simulink model "EGR_CAN"  (R2013b)
settings: Solver=FixedStepDiscrete  StartTime=0.0  StopTime=0.5  FixedStep=Ts  RelTol=1e-3
values from neighbouring files (symbols this model uses):
  C_STEPM_ELEC_TIM_COEFF = Simulink.Parameter    [EGR_CAN_Model_Init.m]
  K_EGR_CAN_ACT_DC_COMP = Simulink.Parameter    [EGR_CAN_Model_Init.m]
  K_EGR_CAN_ACT_POS_MAX = Simulink.Parameter    [EGR_CAN_Model_Init.m]
  K_EGR_CAN_ACT_POS_MIN = Simulink.Parameter    [EGR_CAN_Model_Init.m]
  K_EGR_CAN_TARGET_POS_MAX = Simulink.Parameter    [EGR_CAN_Model_Init.m]
  K_EGR_CAN_TARGET_POS_MIN = Simulink.Parameter    [EGR_CAN_Model_Init.m]
  K_PID_D_TERM = Simulink.Parameter    [EGR_CAN_Model_Init.m]
  K_PID_I_TERM = Simulink.Parameter    [EGR_CAN_Model_Init.m]
  K_PID_P_TERM = Simulink.Parameter    [EGR_CAN_Model_Init.m]
  K_STEPM_DAMPING_COEFF = Simulink.Parameter    [EGR_CAN_Model_Init.m]
  K_STEPM_INERTIA = Simulink.Parameter    [EGR_CAN_Model_Init.m]
  K_STEPM_SELF_DAMPING_COEFF = Simulink.Parameter    [EGR_CAN_Model_Init.m]
  K_STEPM_STEP_NUM = Simulink.Parameter    [EGR_CAN_Model_Init.m]
  K_STEPM_TF = Simulink.Parameter    [EGR_CAN_Model_Init.m]
  Ts = 1e-4    (= 0.0001)    [EGR_CAN_Model_Init.m]
undefined symbols (not defined in the file or in its folder): DiscIntNeverNeededParam
libraries: simulink x1
settings Model: Creator=Administrator  LastModifiedBy=TTI1783
settings OptimizationCC: InlineParams=on  UseFloatMulNetSlope=on  UseSpecifiedMinMax=on  InlineInvariantSignals=on  EnhancedBackFolding=on  ZeroExternalMemoryAtStartup=off  ZeroInternalMemoryAtStartup=off  EfficientFloat2IntCast=on  OptimizeModelRefInitCode=on  LifeSpan=1  MaxStackSize=64
settings DebuggingCC: MergeDetectMultiDrivingBlocksExec=error
settings HardwareCC: ProdLargestAtomicInteger=Long  ProdLargestAtomicFloat=Double  ProdIntDivRoundTo=Floor  ProdEndianess=LittleEndian  ProdHWDeviceType=ARM Compatible->ARM Cortex
settings RTWCC: SystemTargetFile=ert.tlc  GenCodeOnly=on  GenerateMakefile=off  TemplateMakefile=ert_default_tmf  Description=Embedded Coder  GenerateReport=on  ProcessScript=ert_make_rtw_hook  Toolchain=GNU Tools for ARM Embedded Processors  IncludeHyperlinkInReport=on  LaunchReport=on  GenerateTraceInfo=on  GenerateTraceReport=on  GenerateTraceReportSl=on  GenerateTraceReportSf=on  GenerateTraceReportEml=on  RTWCompilerOptimization=On
settings CodeAppCC: ForceParamTrailComments=on  IgnoreCustomStorageClasses=off  OperatorAnnotations=on  SimulinkDataObjDesc=on  SFDataObjDesc=on  MATLABFcnDesc=on  InsertBlockDesc=on  MATLABSourceComments=on  EnableCustomComments=on  ReqsInCode=on
settings ERTTargetCC: CodeReplacementLibrary=ANSI_C  GenerateSampleERTMain=on  IncludeMdlTerminateFcn=off  CombineSignalStateStructs=on  SuppressErrorStatus=on  SupportNonFinite=off  InlinedParameterPlacement=NonHierarchical  ERTCustomFileTemplate=example_file_process.tlc  ConvertIfToSwitch=on  SuppressUnreachableDefaultCases=on

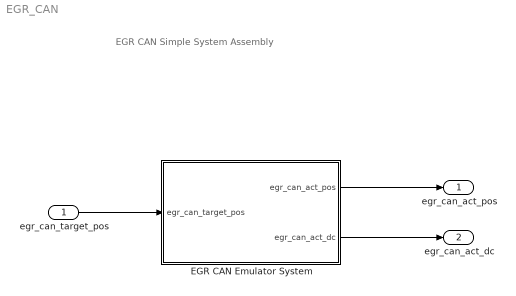
== system EGR_CAN ==
  note: EGR CAN Simple System Assembly
  egr_can_target_pos : Inport
  EGR CAN Emulator System : Subsystem
  egr_can_act_pos : Outport
  egr_can_act_dc : Outport  Port=2
  wires:
  EGR CAN Emulator System/1(egr_can_act_pos) -> egr_can_act_pos/1
  egr_can_target_pos/1 -> EGR CAN Emulator System/1(egr_can_target_pos)
  EGR CAN Emulator System/2(egr_can_act_dc) -> egr_can_act_dc/1

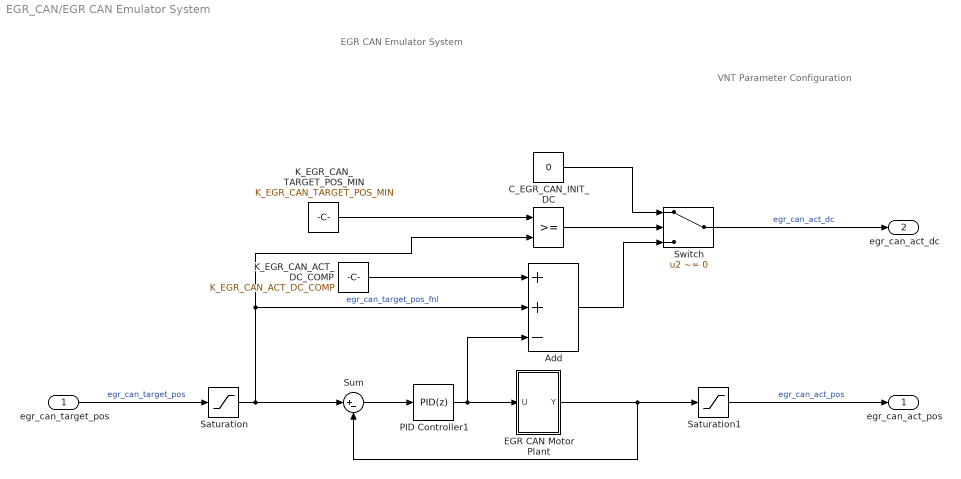
== system EGR_CAN/EGR CAN Emulator System ==
  note: VNT Parameter
      | Configuration
  note: EGR CAN Emulator System
  egr_can_target_pos : Inport
  " " : RelationalOperator  OutDataTypeStr=boolean
  Add : Sum  Inputs=++-
  C_EGR_CAN_INIT_DC : Constant  Value=0
  EGR CAN Motor Plant : Subsystem
  K_EGR_CAN_ACT_DC_COMP : Constant  Value=K_EGR_CAN_ACT_DC_COMP
  K_EGR_CAN_TARGET_POS_MIN : Constant  Value=K_EGR_CAN_TARGET_POS_MIN
  PID Controller1 : simulink/Continuous/PID Controller  Controller=PID  TimeDomain=Discrete-time  SampleTime=Ts  IntegratorMethod=Forward Euler  FilterMethod=Forward Euler  Form=Ideal  P=K_PID_P_TERM  I=K_PID_I_TERM  D=K_PID_D_TERM  N=100  InitialConditionSource=internal  InitialConditionForIntegrator=0  InitialConditionForFilter=0  ExternalReset=none  LimitOutput=off  UpperSaturationLimit=inf  LowerSaturationLimit=-inf  LinearizeAsGain=on  AntiWindupMode=none  Kb=1  TrackingMode=off  Kt=1  PParamMin=[]  PParamMax=[]  IParamMin=[]  IParamMax=[]  DParamMin=[]  DParamMax=[]  NParamMin=[]  NParamMax=[]  KbParamMin=[]  KbParamMax=[]  KtParamMin=[]  KtParamMax=[]  POutMin=[]  POutMax=[]  IOutMin=[]  IOutMax=[]  DOutMin=[]  DOutMax=[]  NOutMin=[]  NOutMax=[]  KbOutMin=[]  KbOutMax=[]  KtOutMin=[]  KtOutMax=[]  IntegratorOutMin=[]  IntegratorOutMax=[]  FilterOutMin=[]  FilterOutMax=[]  SumOutMin=[]  SumOutMax=[]  SumI1OutMin=[]  SumI1OutMax=[]  SumI2OutMin=[]  SumI2OutMax=[]  SumI3OutMin=[]  SumI3OutMax=[]  SumDOutMin=[]  SumDOutMax=[]  SaturationOutMin=[]  SaturationOutMax=[]  IntegratorContinuousStateAttributes=''  IntegratorStateMustResolveToSignalObject=off  IntegratorRTWStateStorageClass=Auto  FilterContinuousStateAttributes=''  FilterStateMustResolveToSignalObject=off  FilterRTWStateStorageClass=Auto
  Saturation : Saturate  UpperLimit=K_EGR_CAN_TARGET_POS_MAX  LowerLimit=K_EGR_CAN_TARGET_POS_MIN
  Saturation1 : Saturate  UpperLimit=K_EGR_CAN_ACT_POS_MAX  LowerLimit=K_EGR_CAN_ACT_POS_MIN
  Sum : Sum  Inputs=|+-
  Switch : Switch  Criteria=u2 ~= 0
  egr_can_act_pos : Outport
  egr_can_act_dc : Outport  Port=2
  wires:
  egr_can_target_pos/1 -> Saturation/1  "egr_can_target_pos"
  PID Controller1/1 -> Add/3, EGR CAN Motor Plant/1(U)
  Sum/1 -> PID Controller1/1
  Saturation1/1 -> egr_can_act_pos/1  "egr_can_act_pos"
  EGR CAN Motor Plant/1(Y) -> Saturation1/1, Sum/2
  Saturation/1 -> Add/2, " "/2, Sum/1  "egr_can_target_pos_fnl"
  K_EGR_CAN_ACT_DC_COMP/1 -> Add/1
  Add/1 -> Switch/3
  Switch/1 -> egr_can_act_dc/1  "egr_can_act_dc"
  " "/1 -> Switch/2
  C_EGR_CAN_INIT_DC/1 -> Switch/1
  K_EGR_CAN_TARGET_POS_MIN/1 -> " "/1

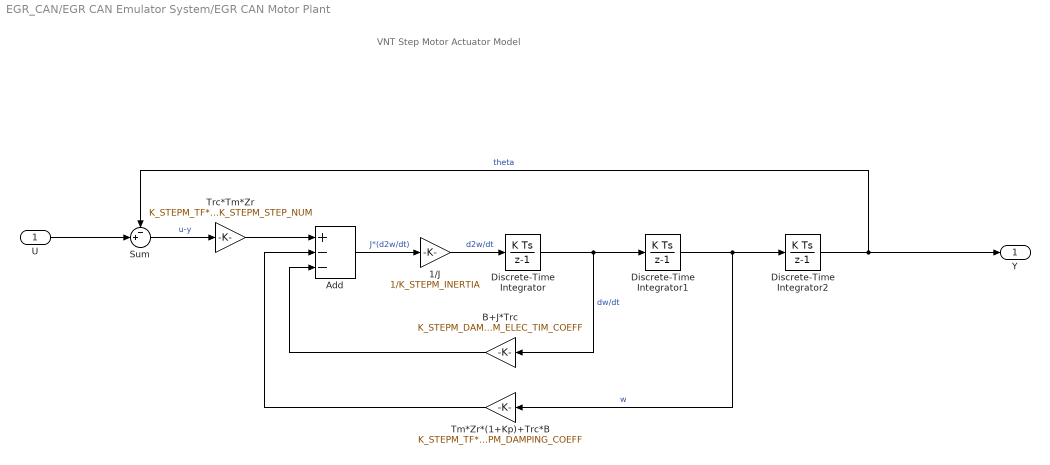
== system EGR_CAN/EGR CAN Emulator System/EGR CAN Motor Plant ==
  note: VNT Step Motor Actuator Model
  U : Inport
  1/J : Gain  Gain=1/K_STEPM_INERTIA
  Add : Sum  Inputs=+--
  B+J*Trc : Gain  Gain=K_STEPM_DAMPING_COEFF+K_STEPM_INERTIA*C_STEPM_ELEC_TIM_COEFF
  Discrete-Time Integrator : DiscreteIntegrator  SampleTime=Ts  ICPrevOutput=DiscIntNeverNeededParam  ICPrevScaledInput=DiscIntNeverNeededParam
  Discrete-Time Integrator1 : DiscreteIntegrator  SampleTime=Ts  ICPrevOutput=DiscIntNeverNeededParam  ICPrevScaledInput=DiscIntNeverNeededParam
  Discrete-Time Integrator2 : DiscreteIntegrator  SampleTime=Ts  ICPrevOutput=DiscIntNeverNeededParam  ICPrevScaledInput=DiscIntNeverNeededParam
  Sum : Sum  Inputs=-+|
  Tm*Zr*(1+Kp)+Trc*B : Gain  Gain=K_STEPM_TF*K_STEPM_STEP_NUM*(1+K_STEPM_SELF_DAMPING_COEFF)+C_STEPM_ELEC_TIM_COEFF*K_STEPM_DAMPING_COEFF
  Trc*Tm*Zr : Gain  Gain=K_STEPM_TF*C_STEPM_ELEC_TIM_COEFF*K_STEPM_STEP_NUM
  Y : Outport
  wires:
  B+J*Trc/1 -> Add/3
  Add/1 -> 1/J/1  "J*(d2w/dt)"
  Trc*Tm*Zr/1 -> Add/1
  Tm*Zr*(1+Kp)+Trc*B/1 -> Add/2
  U/1 -> Sum/2
  Discrete-Time Integrator2/1 -> Y/1, Sum/1  "theta"
  Sum/1 -> Trc*Tm*Zr/1  "u-y"
  Discrete-Time Integrator/1 -> Discrete-Time Integrator1/1, B+J*Trc/1  "dw/dt"
  1/J/1 -> Discrete-Time Integrator/1  "d2w/dt"
  Discrete-Time Integrator1/1 -> Discrete-Time Integrator2/1, Tm*Zr*(1+Kp)+Trc*B/1  "w"
